simulink model "cont_dis_regler_2"  (Simulink 7.6)
settings: Solver=ode45  StartTime=0.0  StopTime=10  RelTol=1e-3
values from neighbouring files (symbols this model uses):
  a_0 = T_1/T_2*exp(-T_a*(1/T_2-1/T_1))    [koeff.m]
  a_1 = T_1/T_2*exp(-T_a/T_2)    [koeff.m]
  b_1 = exp(-T_a/T_2)    [koeff.m]
undefined symbols (not defined in the file or in its folder): k, T_1, T_2, T_w, x_c
settings Model: Creator=akoerner  LastModifiedBy=Stuffy
settings DebuggingCC: SaveWithParameterizedLinksMsg=none  StrictBusMsg=Warning

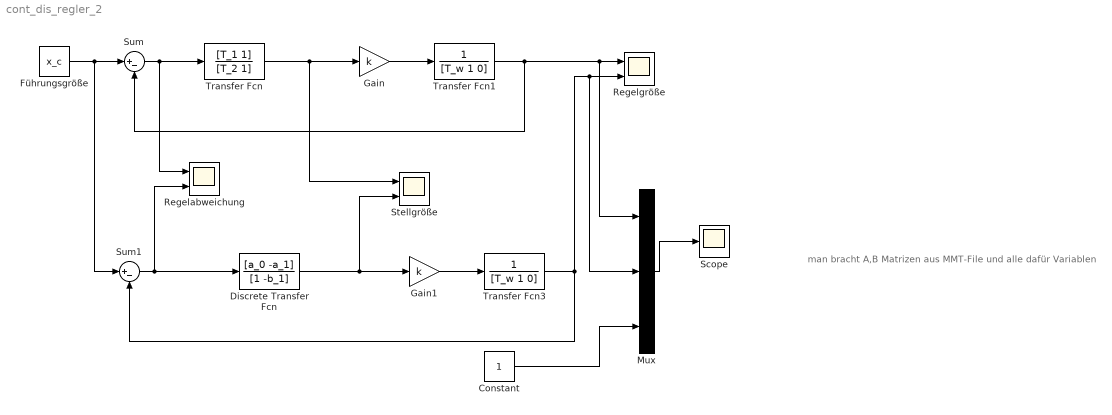
== system cont_dis_regler_2 ==
  note: man bracht A,B Matrizen aus MMT-File
      | und alle dafür Variablen
  Constant : Constant
  Discrete Transfer Fcn : DiscreteTransferFcn  Numerator=[a_0 -a_1]  Denominator=[1 -b_1]  SampleTime=0.2
  Führungsgröße : Constant  Value=x_c
  Gain : Gain  Gain=k
  Gain1 : Gain  Gain=k
  Mux : Mux  Inputs=3
  Regelabweichung : Scope  NumInputPorts=2
      settings: YMin=-5~-5  YMax=5~5  SaveName=ScopeData2
  Regelgröße : Scope  NumInputPorts=2
      settings: YMin=-5~-5  YMax=5~5
  Scope : Scope
  Stellgröße : Scope  NumInputPorts=2
      settings: YMin=-5~-5  YMax=5~5  SaveName=ScopeData3
  Sum : Sum  Inputs=|+-
  Sum1 : Sum  Inputs=|+-
  Transfer Fcn : TransferFcn  Numerator=[T_1 1]  Denominator=[T_2 1]
  Transfer Fcn1 : TransferFcn  Denominator=[T_w 1 0]
  Transfer Fcn3 : TransferFcn  Denominator=[T_w 1 0]
  wires:
  Sum/1 -> Transfer Fcn/1, Regelabweichung/1
  Transfer Fcn/1 -> Gain/1, Stellgröße/1
  Gain/1 -> Transfer Fcn1/1
  Transfer Fcn1/1 -> Sum/2, Regelgröße/1, Mux/1
  Führungsgröße/1 -> Sum/1, Sum1/1
  Gain1/1 -> Transfer Fcn3/1
  Transfer Fcn3/1 -> Sum1/2, Regelgröße/2, Mux/2
  Discrete Transfer Fcn/1 -> Gain1/1, Stellgröße/2
  Sum1/1 -> Discrete Transfer Fcn/1, Regelabweichung/2
  Mux/1 -> Scope/1
  Constant/1 -> Mux/3
